simulink subsystem "rss_ComFaltDia"  (R2023a)
settings: Solver=VariableStepAuto  StartTime=0.0  StopTime=10.0  RelTol=1e-3
undefined symbols (not defined in the file): Cdbl_nMechSpdMaxVal, Cdbl_numComFramLosSmpNum, Cdbl_numDataExcdLimSmpNum, ENM_TYPE_FALT, Gs16_nMaxRefMechSpd_C, Gu16_ctComLosFaltConfCnt_C, Gu16_ctComLosFaltRcvyCnt_C, Gu16_ctComRolCntFaltConfCnt_C, Gu16_ctComRolCntFaltRcvyCnt_C, Gu16_ctCRCFaltConfCnt_C, Gu16_ctCRCFaltRcvyCnt_C, Gu16_ctMesgLngthFaltConfCnt_C, Gu16_ctMesgLngthFaltRcvyCnt_C, Gu8_ctComFramLosFaltJudgCnt_C, Gu8_ctDataExcdLimFaltJudgCnt_C, Gu8_RollingMax_C, Gu8_RollingMin_C
libraries: lib_debounce x7, simulink x5, lib_conversion x2, lib_fault_definiteness x1
settings Model: Creator=xiaoqiang.yuan  LastModifiedBy=xiaoqiang.yuan

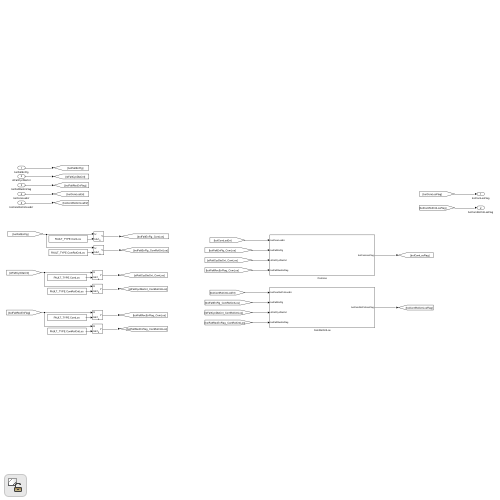
[thumbnail: Simulink's stored preview of the top-level diagram]
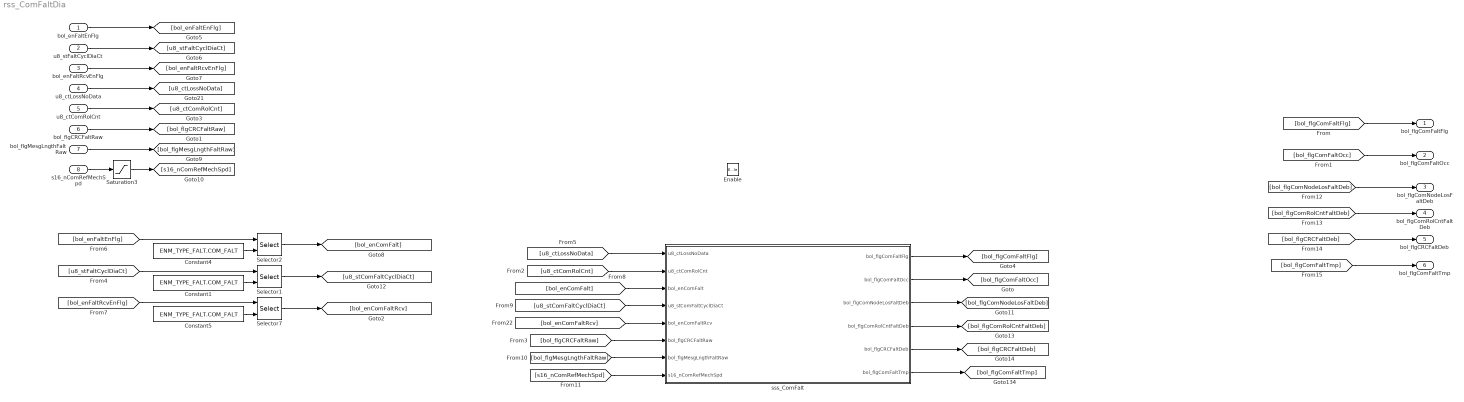
== system rss_ComFaltDia ==
  bol_enFaltEnFlg : Inport  OutDataTypeStr=boolean
  u8_stFaltCyclDiaCt : Inport  Port=2  OutDataTypeStr=uint8
  bol_enFaltRcvEnFlg : Inport  Port=3  OutDataTypeStr=boolean
  u8_ctLossNoData : Inport  Port=4  OutDataTypeStr=uint8
  u8_ctComRolCnt : Inport  Port=5  OutDataTypeStr=uint8
  bol_flgCRCFaltRaw : Inport  Port=6  OutDataTypeStr=boolean
  bol_flgMesgLngthFaltRaw : Inport  Port=7  OutDataTypeStr=boolean
  s16_nComRefMechSpd : Inport  Port=8  OutDataTypeStr=dt_Standardize_s16p15b0
  Enable : EnablePort
  Constant1 : Constant  Value=ENM_TYPE_FALT.COM_FALT
  Constant4 : Constant  Value=ENM_TYPE_FALT.COM_FALT
  Constant5 : Constant  Value=ENM_TYPE_FALT.COM_FALT
  Saturation3 : Saturate  UpperLimit=Cdbl_nMechSpdMaxVal  LowerLimit=-Cdbl_nMechSpdMaxVal
  Selector1 : Selector  IndexMode=Zero-based  InputPortWidth=Cdbl_numFaltDiaNum  IndexOptions=Index vector (port)  Indices=[1 3]  OutputSizes=1
  Selector2 : Selector  IndexMode=Zero-based  InputPortWidth=Cdbl_numFaltDiaNum  IndexOptions=Index vector (port)  Indices=[1 3]  OutputSizes=1
  Selector7 : Selector  IndexMode=Zero-based  InputPortWidth=Cdbl_numFaltDiaNum  IndexOptions=Index vector (port)  Indices=[1 3]  OutputSizes=1
  sss_ComFalt : Subsystem
  bol_flgComFaltFlg : Outport  OutDataTypeStr=boolean
  bol_flgComFaltOcc : Outport  Port=2  OutDataTypeStr=boolean
  bol_flgComNodeLosFaltDeb : Outport  Port=3  OutDataTypeStr=boolean
  bol_flgComRolCntFaltDeb : Outport  Port=4  OutDataTypeStr=boolean
  bol_flgCRCFaltDeb : Outport  Port=5  OutDataTypeStr=boolean
  bol_flgComFaltTmp : Outport  Port=6  OutDataTypeStr=boolean
  wires:
  [bol_flgComFaltFlg] -> bol_flgComFaltFlg/1
  [bol_flgComFaltOcc] -> bol_flgComFaltOcc/1
  [u8_stFaltCyclDiaCt] -> Selector1/1
  [bol_enFaltEnFlg] -> Selector2/1
  bol_enFaltEnFlg/1 -> [bol_enFaltEnFlg]
  bol_enFaltRcvEnFlg/1 -> [bol_enFaltRcvEnFlg]
  [u8_ctLossNoData] -> sss_ComFalt/1(u8_ctLossNoData)
  Constant1/1 -> Selector1/2
  [u8_stComFaltCyclDiaCt] -> sss_ComFalt/4(u8_stComFaltCyclDiaCt)
  [bol_enComFalt] -> sss_ComFalt/3(bol_enComFalt)
  Constant4/1 -> Selector2/2
  Constant5/1 -> Selector7/2
  Selector1/1 -> [u8_stComFaltCyclDiaCt]
  u8_ctLossNoData/1 -> [u8_ctLossNoData]
  Selector7/1 -> [bol_enComFaltRcv]
  [bol_enFaltRcvEnFlg] -> Selector7/1
  Selector2/1 -> [bol_enComFalt]
  [bol_enComFaltRcv] -> sss_ComFalt/5(bol_enComFaltRcv)
  u8_stFaltCyclDiaCt/1 -> [u8_stFaltCyclDiaCt]
  sss_ComFalt/1(bol_flgComFaltFlg) -> [bol_flgComFaltFlg]
  u8_ctComRolCnt/1 -> [u8_ctComRolCnt]
  [u8_ctComRolCnt] -> sss_ComFalt/2(u8_ctComRolCnt)
  sss_ComFalt/2(bol_flgComFaltOcc) -> [bol_flgComFaltOcc]
  bol_flgCRCFaltRaw/1 -> [bol_flgCRCFaltRaw]
  bol_flgMesgLngthFaltRaw/1 -> [bol_flgMesgLngthFaltRaw]
  s16_nComRefMechSpd/1 -> Saturation3/1
  [bol_flgCRCFaltRaw] -> sss_ComFalt/6(bol_flgCRCFaltRaw)
  [bol_flgMesgLngthFaltRaw] -> sss_ComFalt/7(bol_flgMesgLngthFaltRaw)
  [s16_nComRefMechSpd] -> sss_ComFalt/8(s16_nComRefMechSpd)
  Saturation3/1 -> [s16_nComRefMechSpd]
  [bol_flgCRCFaltDeb] -> bol_flgCRCFaltDeb/1
  [bol_flgComRolCntFaltDeb] -> bol_flgComRolCntFaltDeb/1
  [bol_flgComNodeLosFaltDeb] -> bol_flgComNodeLosFaltDeb/1
  sss_ComFalt/5(bol_flgCRCFaltDeb) -> [bol_flgCRCFaltDeb]
  sss_ComFalt/4(bol_flgComRolCntFaltDeb) -> [bol_flgComRolCntFaltDeb]
  sss_ComFalt/3(bol_flgComNodeLosFaltDeb) -> [bol_flgComNodeLosFaltDeb]
  [bol_flgComFaltTmp] -> bol_flgComFaltTmp/1
  sss_ComFalt/6(bol_flgComFaltTmp) -> [bol_flgComFaltTmp]

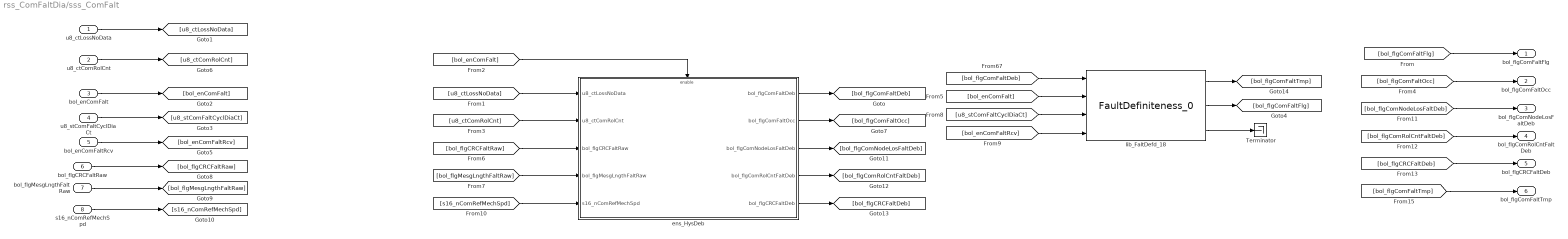
== system rss_ComFaltDia/sss_ComFalt ==
  u8_ctLossNoData : Inport
  u8_ctComRolCnt : Inport  Port=2
  bol_enComFalt : Inport  Port=3
  u8_stComFaltCyclDiaCt : Inport  Port=4
  bol_enComFaltRcv : Inport  Port=5
  bol_flgCRCFaltRaw : Inport  Port=6
  bol_flgMesgLngthFaltRaw : Inport  Port=7
  s16_nComRefMechSpd : Inport  Port=8
  Terminator : Terminator
  ens_HysDeb : Subsystem  Variant=on  VariantControlMode=label  VariantControl=Choice  LabelModeActiveChoice=GEELY_PROJECT
  lib_FaltDefd_18 : lib_fault_definiteness/FaultDefiniteness_0  lb_FaltWaitRecvCnt=0
  bol_flgComFaltFlg : Outport
  bol_flgComFaltOcc : Outport  Port=2
  bol_flgComNodeLosFaltDeb : Outport  Port=3
  bol_flgComRolCntFaltDeb : Outport  Port=4
  bol_flgCRCFaltDeb : Outport  Port=5
  bol_flgComFaltTmp : Outport  Port=6
  wires:
  [bol_flgComFaltTmp] -> bol_flgComFaltTmp/1
  ens_HysDeb/5(bol_flgCRCFaltDeb) -> [bol_flgCRCFaltDeb]
  ens_HysDeb/4(bol_flgComRolCntFaltDeb) -> [bol_flgComRolCntFaltDeb]
  ens_HysDeb/3(bol_flgComNodeLosFaltDeb) -> [bol_flgComNodeLosFaltDeb]
  [bol_flgCRCFaltDeb] -> bol_flgCRCFaltDeb/1
  [bol_flgComRolCntFaltDeb] -> bol_flgComRolCntFaltDeb/1
  [bol_flgComNodeLosFaltDeb] -> bol_flgComNodeLosFaltDeb/1
  ens_HysDeb/2(bol_flgComFaltOcc) -> [bol_flgComFaltOcc]
  ens_HysDeb/1(bol_flgComFaltDeb) -> [bol_flgComFaltDeb]
  [bol_enComFalt] -> ens_HysDeb/Enable
  [s16_nComRefMechSpd] -> ens_HysDeb/5(s16_nComRefMechSpd)
  [bol_flgMesgLngthFaltRaw] -> ens_HysDeb/4(bol_flgMesgLngthFaltRaw)
  [bol_flgCRCFaltRaw] -> ens_HysDeb/3(bol_flgCRCFaltRaw)
  [u8_ctComRolCnt] -> ens_HysDeb/2(u8_ctComRolCnt)
  [u8_ctLossNoData] -> ens_HysDeb/1(u8_ctLossNoData)
  bol_flgMesgLngthFaltRaw/1 -> [bol_flgMesgLngthFaltRaw]
  s16_nComRefMechSpd/1 -> [s16_nComRefMechSpd]
  bol_flgCRCFaltRaw/1 -> [bol_flgCRCFaltRaw]
  [bol_flgComFaltOcc] -> bol_flgComFaltOcc/1
  u8_ctComRolCnt/1 -> [u8_ctComRolCnt]
  lib_FaltDefd_18/1 -> [bol_flgComFaltTmp]
  lib_FaltDefd_18/2 -> [bol_flgComFaltFlg]
  lib_FaltDefd_18/3 -> Terminator/1
  bol_enComFaltRcv/1 -> [bol_enComFaltRcv]
  u8_stComFaltCyclDiaCt/1 -> [u8_stComFaltCyclDiaCt]
  bol_enComFalt/1 -> [bol_enComFalt]
  [bol_flgComFaltFlg] -> bol_flgComFaltFlg/1
  u8_ctLossNoData/1 -> [u8_ctLossNoData]
  [bol_enComFaltRcv] -> lib_FaltDefd_18/4
  [u8_stComFaltCyclDiaCt] -> lib_FaltDefd_18/3
  [bol_enComFalt] -> lib_FaltDefd_18/2
  [bol_flgComFaltDeb] -> lib_FaltDefd_18/1

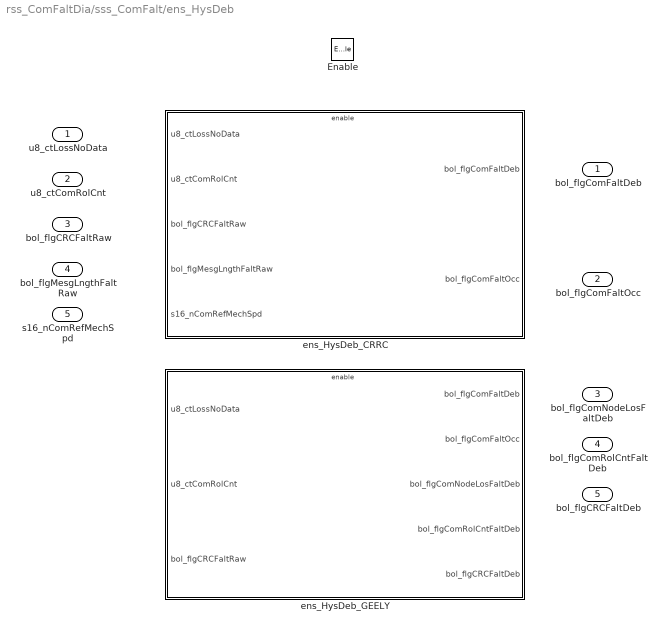
== system rss_ComFaltDia/sss_ComFalt/ens_HysDeb ==
  u8_ctLossNoData : Inport
  u8_ctComRolCnt : Inport  Port=2
  bol_flgCRCFaltRaw : Inport  Port=3
  bol_flgMesgLngthFaltRaw : Inport  Port=4
  s16_nComRefMechSpd : Inport  Port=5
  Enable : EnablePort
  ens_HysDeb_CRRC : Subsystem  VariantControl=CRRC_PROJECT
  ens_HysDeb_GEELY : Subsystem  VariantControl=GEELY_PROJECT
  bol_flgComFaltDeb : Outport
  bol_flgComFaltOcc : Outport  Port=2
  bol_flgComNodeLosFaltDeb : Outport  Port=3
  bol_flgComRolCntFaltDeb : Outport  Port=4
  bol_flgCRCFaltDeb : Outport  Port=5

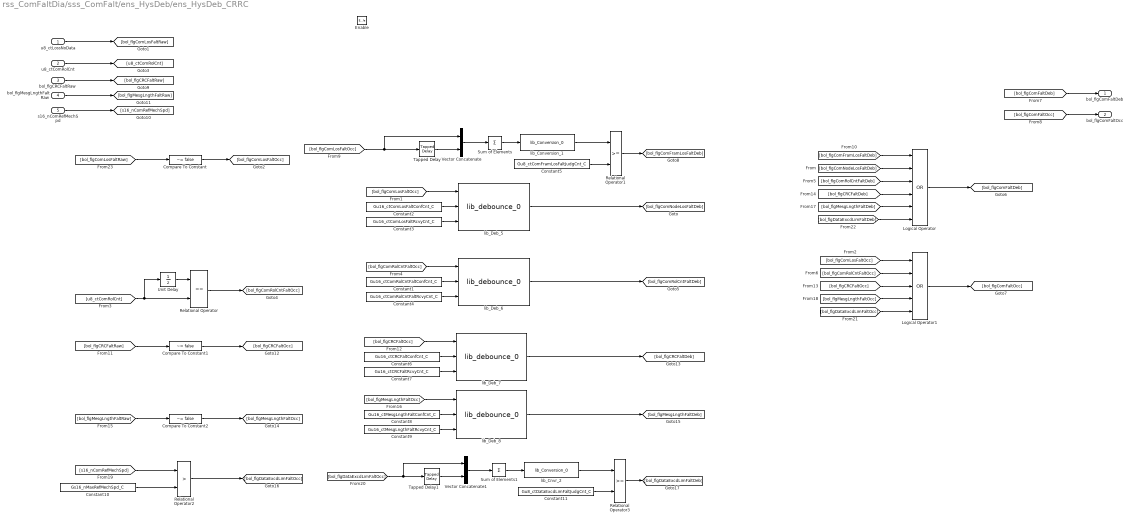
== system rss_ComFaltDia/sss_ComFalt/ens_HysDeb/ens_HysDeb_CRRC ==
  u8_ctLossNoData : Inport
  u8_ctComRolCnt : Inport  Port=2
  bol_flgCRCFaltRaw : Inport  Port=3
  bol_flgMesgLngthFaltRaw : Inport  Port=4
  s16_nComRefMechSpd : Inport  Port=5
  Enable : EnablePort
  Compare To Constant : simulink/Logic and Bit Operations/Compare To Constant  relop=~=  const=false  OutDataTypeStr=boolean
  Compare To Constant1 : simulink/Logic and Bit Operations/Compare To Constant  relop=~=  const=false  OutDataTypeStr=boolean
  Compare To Constant2 : simulink/Logic and Bit Operations/Compare To Constant  relop=~=  const=false  OutDataTypeStr=boolean
  Constant1 : Constant  Value=Gu16_ctComRolCntFaltConfCnt_C
  Constant10 : Constant  Value=Gs16_nMaxRefMechSpd_C
  Constant11 : Constant  Value=Gu8_ctDataExcdLimFaltJudgCnt_C
  Constant2 : Constant  Value=Gu16_ctComLosFaltConfCnt_C
  Constant3 : Constant  Value=Gu16_ctComLosFaltRcvyCnt_C
  Constant4 : Constant  Value=Gu16_ctComRolCntFaltRcvyCnt_C
  Constant5 : Constant  Value=Gu8_ctComFramLosFaltJudgCnt_C
  Constant6 : Constant  Value=Gu16_ctCRCFaltConfCnt_C
  Constant7 : Constant  Value=Gu16_ctCRCFaltRcvyCnt_C
  Constant8 : Constant  Value=Gu16_ctMesgLngthFaltConfCnt_C
  Constant9 : Constant  Value=Gu16_ctMesgLngthFaltRcvyCnt_C
  Logical Operator : Logic  Operator=OR  Inputs=6  AllPortsSameDT=off  OutDataTypeStr=boolean
  Logical Operator1 : Logic  Operator=OR  Inputs=5  AllPortsSameDT=off  OutDataTypeStr=boolean
  Relational Operator : RelationalOperator  Operator===  OutDataTypeStr=boolean  RndMeth=Simplest  InputSameDT=off
  Relational Operator1 : RelationalOperator  OutDataTypeStr=boolean  RndMeth=Simplest  InputSameDT=off
  Relational Operator2 : RelationalOperator  Operator=>  OutDataTypeStr=boolean  RndMeth=Simplest  InputSameDT=off
  Relational Operator3 : RelationalOperator  OutDataTypeStr=boolean  RndMeth=Simplest  InputSameDT=off
  Sum of Elements : Sum  Inputs=+  OutDataTypeStr=Inherit: Inherit via back propagation  RndMeth=Simplest
  Sum of Elements1 : Sum  Inputs=+  OutDataTypeStr=Inherit: Inherit via back propagation  RndMeth=Simplest
  Tapped Delay : simulink/Discrete/Tapped Delay  vinit=0  samptime=-1  NumDelays=Cdbl_numComFramLosSmpNum-1  DelayOrder=Oldest  includeCurrent=off
  Tapped Delay1 : simulink/Discrete/Tapped Delay  vinit=0  samptime=-1  NumDelays=Cdbl_numDataExcdLimSmpNum-1  DelayOrder=Oldest  includeCurrent=off
  Unit Delay : UnitDelay  SampleTime=-1  HasFrameUpgradeWarning=on
  Vector Concatenate : Concatenate
  Vector Concatenate1 : Concatenate
  lib_Cnvr_2 : lib_conversion/lib_Conversion_0  lb_parDataType=uint8  lb_parOutpMaxVal=[]  lb_parOutpMinVal=[]  lb_parSatFlag=off
  lib_Conversion_1 : lib_conversion/lib_Conversion_0  lb_parDataType=uint8  lb_parOutpMaxVal=[]  lb_parOutpMinVal=[]  lb_parSatFlag=off
  lib_Deb_{5..8} (4 alike) : lib_debounce/lib_debounce_0
  bol_flgComFaltDeb : Outport
  bol_flgComFaltOcc : Outport  Port=2
  wires:
  [bol_flgDataExcdLimFaltOcc] -> Logical Operator1/5
  [bol_flgMesgLngthFaltOcc] -> Logical Operator1/4
  [bol_flgDataExcdLimFaltDeb] -> Logical Operator/6
  [bol_flgMesgLngthFaltDeb] -> Logical Operator/5
  Relational Operator3/1 -> [bol_flgDataExcdLimFaltDeb]
  Constant11/1 -> Relational Operator3/2
  lib_Cnvr_2/1 -> Relational Operator3/1
  Tapped Delay1/1 -> Vector Concatenate1/2
  Vector Concatenate1/1 -> Sum of Elements1/1
  [bol_flgDataExcdLimFaltOcc] -> Tapped Delay1/1, Vector Concatenate1/1
  Sum of Elements1/1 -> lib_Cnvr_2/1
  Relational Operator2/1 -> [bol_flgDataExcdLimFaltOcc]
  Constant10/1 -> Relational Operator2/2
  [s16_nComRefMechSpd] -> Relational Operator2/1
  lib_Deb_8/1 -> [bol_flgMesgLngthFaltDeb]
  [bol_flgMesgLngthFaltOcc] -> lib_Deb_8/1
  Constant8/1 -> lib_Deb_8/2
  Constant9/1 -> lib_Deb_8/3
  Compare To Constant2/1 -> [bol_flgMesgLngthFaltOcc]
  [bol_flgMesgLngthFaltRaw] -> Compare To Constant2/1
  [bol_flgCRCFaltOcc] -> Logical Operator1/3
  [bol_flgComRolCntFaltOcc] -> Logical Operator1/2
  [bol_flgComLosFaltOcc] -> Logical Operator1/1
  [bol_flgComFramLosFaltDeb] -> Logical Operator/1
  [bol_flgComNodeLosFaltDeb] -> Logical Operator/2
  [bol_flgComRolCntFaltDeb] -> Logical Operator/3
  [bol_flgCRCFaltDeb] -> Logical Operator/4
  lib_Deb_7/1 -> [bol_flgCRCFaltDeb]
  Constant7/1 -> lib_Deb_7/3
  Constant6/1 -> lib_Deb_7/2
  [bol_flgCRCFaltOcc] -> lib_Deb_7/1
  Compare To Constant1/1 -> [bol_flgCRCFaltOcc]
  [bol_flgCRCFaltRaw] -> Compare To Constant1/1
  s16_nComRefMechSpd/1 -> [s16_nComRefMechSpd]
  bol_flgCRCFaltRaw/1 -> [bol_flgCRCFaltRaw]
  bol_flgMesgLngthFaltRaw/1 -> [bol_flgMesgLngthFaltRaw]
  Relational Operator1/1 -> [bol_flgComFramLosFaltDeb]
  Constant5/1 -> Relational Operator1/2
  lib_Conversion_1/1 -> Relational Operator1/1
  Sum of Elements/1 -> lib_Conversion_1/1
  [bol_flgComLosFaltOcc] -> Tapped Delay/1, Vector Concatenate/1
  Tapped Delay/1 -> Vector Concatenate/2
  Vector Concatenate/1 -> Sum of Elements/1
  [bol_flgComFaltOcc] -> bol_flgComFaltOcc/1
  Logical Operator1/1 -> [bol_flgComFaltOcc]
  Logical Operator/1 -> [bol_flgComFaltDeb]
  lib_Deb_6/1 -> [bol_flgComRolCntFaltDeb]
  [bol_flgComRolCntFaltOcc] -> lib_Deb_6/1
  Constant1/1 -> lib_Deb_6/2
  Constant4/1 -> lib_Deb_6/3
  Relational Operator/1 -> [bol_flgComRolCntFaltOcc]
  Unit Delay/1 -> Relational Operator/1
  [u8_ctComRolCnt] -> Unit Delay/1, Relational Operator/2
  u8_ctComRolCnt/1 -> [u8_ctComRolCnt]
  [bol_flgComLosFaltOcc] -> lib_Deb_5/1
  Compare To Constant/1 -> [bol_flgComLosFaltOcc]
  [bol_flgComLosFaltRaw] -> Compare To Constant/1
  lib_Deb_5/1 -> [bol_flgComNodeLosFaltDeb]
  u8_ctLossNoData/1 -> [bol_flgComLosFaltRaw]
  [bol_flgComFaltDeb] -> bol_flgComFaltDeb/1
  Constant3/1 -> lib_Deb_5/3
  Constant2/1 -> lib_Deb_5/2

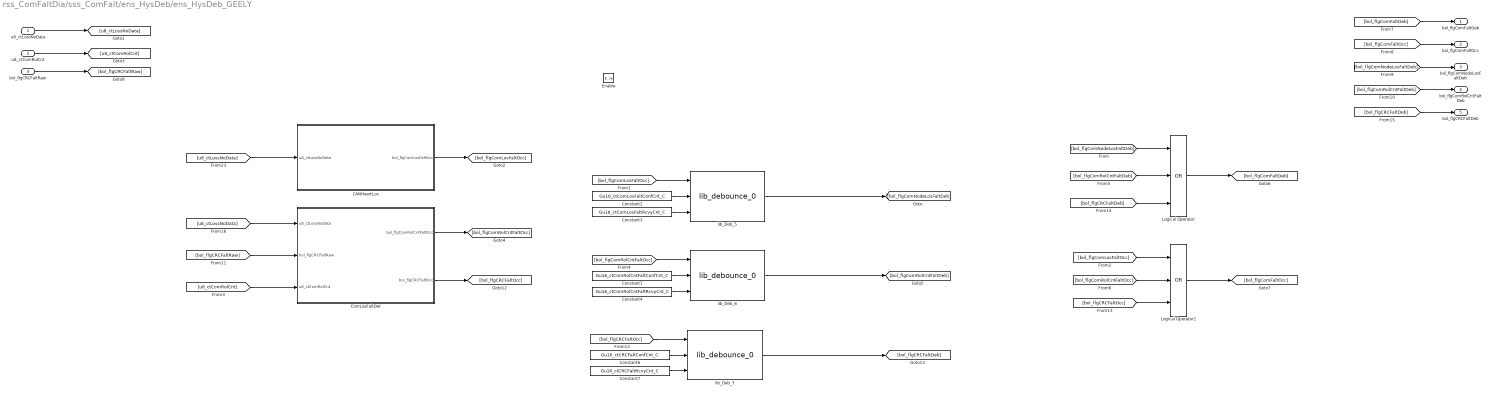
== system rss_ComFaltDia/sss_ComFalt/ens_HysDeb/ens_HysDeb_GEELY ==
  u8_ctLossNoData : Inport
  u8_ctComRolCnt : Inport  Port=2
  bol_flgCRCFaltRaw : Inport  Port=3
  Enable : EnablePort
  CANHeartLos : Subsystem  RTWFcnName=CANHeartLosCheck
      settings: RTWSystemCode=Nonreusable function  RTWFcnNameOpts=User specified
  ComLosFaltDet : Subsystem
  Constant1 : Constant  Value=Gu16_ctComRolCntFaltConfCnt_C
  Constant2 : Constant  Value=Gu16_ctComLosFaltConfCnt_C
  Constant3 : Constant  Value=Gu16_ctComLosFaltRcvyCnt_C
  Constant4 : Constant  Value=Gu16_ctComRolCntFaltRcvyCnt_C
  Constant6 : Constant  Value=Gu16_ctCRCFaltConfCnt_C
  Constant7 : Constant  Value=Gu16_ctCRCFaltRcvyCnt_C
  Logical Operator : Logic  Operator=OR  Inputs=3  AllPortsSameDT=off  OutDataTypeStr=boolean
  Logical Operator1 : Logic  Operator=OR  Inputs=3  AllPortsSameDT=off  OutDataTypeStr=boolean
  lib_Deb_5 : lib_debounce/lib_debounce_0
  lib_Deb_6 : lib_debounce/lib_debounce_0
  lib_Deb_7 : lib_debounce/lib_debounce_0
  bol_flgComFaltDeb : Outport
  bol_flgComFaltOcc : Outport  Port=2
  bol_flgComNodeLosFaltDeb : Outport  Port=3
  bol_flgComRolCntFaltDeb : Outport  Port=4
  bol_flgCRCFaltDeb : Outport  Port=5
  wires:
  [u8_ctLossNoData] -> ComLosFaltDet/1(u8_ctLossNoData)
  CANHeartLos/1(bol_flgComLosFaltOcc) -> [bol_flgComLosFaltOcc]
  [u8_ctLossNoData] -> CANHeartLos/1(u8_ctLossNoData)
  ComLosFaltDet/1(bol_flgComRolCntFaltOcc) -> [bol_flgComRolCntFaltOcc]
  ComLosFaltDet/2(bol_flgCRCFaltOcc) -> [bol_flgCRCFaltOcc]
  [bol_flgCRCFaltRaw] -> ComLosFaltDet/2(bol_flgCRCFaltRaw)
  [u8_ctComRolCnt] -> ComLosFaltDet/3(u8_ctComRolCnt)
  [bol_flgCRCFaltDeb] -> bol_flgCRCFaltDeb/1
  [bol_flgComRolCntFaltDeb] -> bol_flgComRolCntFaltDeb/1
  [bol_flgComNodeLosFaltDeb] -> bol_flgComNodeLosFaltDeb/1
  [bol_flgCRCFaltOcc] -> Logical Operator1/3
  [bol_flgComRolCntFaltOcc] -> Logical Operator1/2
  [bol_flgComLosFaltOcc] -> Logical Operator1/1
  [bol_flgComNodeLosFaltDeb] -> Logical Operator/1
  [bol_flgComRolCntFaltDeb] -> Logical Operator/2
  [bol_flgCRCFaltDeb] -> Logical Operator/3
  lib_Deb_7/1 -> [bol_flgCRCFaltDeb]
  Constant7/1 -> lib_Deb_7/3
  Constant6/1 -> lib_Deb_7/2
  [bol_flgCRCFaltOcc] -> lib_Deb_7/1
  bol_flgCRCFaltRaw/1 -> [bol_flgCRCFaltRaw]
  [bol_flgComFaltOcc] -> bol_flgComFaltOcc/1
  Logical Operator1/1 -> [bol_flgComFaltOcc]
  Logical Operator/1 -> [bol_flgComFaltDeb]
  lib_Deb_6/1 -> [bol_flgComRolCntFaltDeb]
  [bol_flgComRolCntFaltOcc] -> lib_Deb_6/1
  Constant1/1 -> lib_Deb_6/2
  Constant4/1 -> lib_Deb_6/3
  u8_ctComRolCnt/1 -> [u8_ctComRolCnt]
  [bol_flgComLosFaltOcc] -> lib_Deb_5/1
  lib_Deb_5/1 -> [bol_flgComNodeLosFaltDeb]
  u8_ctLossNoData/1 -> [u8_ctLossNoData]
  [bol_flgComFaltDeb] -> bol_flgComFaltDeb/1
  Constant3/1 -> lib_Deb_5/3
  Constant2/1 -> lib_Deb_5/2

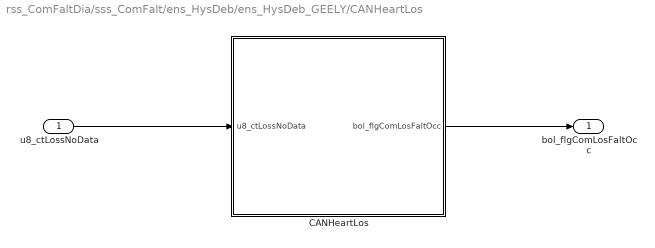
== system rss_ComFaltDia/sss_ComFalt/ens_HysDeb/ens_HysDeb_GEELY/CANHeartLos ==
  u8_ctLossNoData : Inport
  CANHeartLos : Subsystem
  bol_flgComLosFaltOcc : Outport
  wires:
  CANHeartLos/1(bol_flgComLosFaltOcc) -> bol_flgComLosFaltOcc/1
  u8_ctLossNoData/1 -> CANHeartLos/1(u8_ctLossNoData)

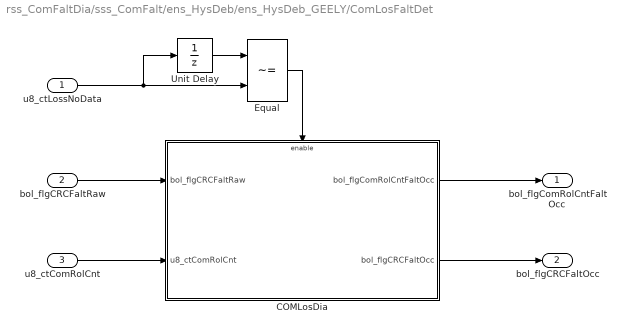
== system rss_ComFaltDia/sss_ComFalt/ens_HysDeb/ens_HysDeb_GEELY/ComLosFaltDet ==
  u8_ctLossNoData : Inport
  bol_flgCRCFaltRaw : Inport  Port=2
  u8_ctComRolCnt : Inport  Port=3
  COMLosDia : Subsystem  TreatAsAtomicUnit=on  RTWFcnName=CANSigLosCheck
      settings: RTWSystemCode=Nonreusable function  RTWFcnNameOpts=User specified
  Equal : RelationalOperator  Operator=~=  OutDataTypeStr=boolean  RndMeth=Simplest  InputSameDT=off
  Unit Delay : UnitDelay  SampleTime=-1  HasFrameUpgradeWarning=on
  bol_flgComRolCntFaltOcc : Outport
  bol_flgCRCFaltOcc : Outport  Port=2
  wires:
  u8_ctLossNoData/1 -> Equal/2, Unit Delay/1
  Unit Delay/1 -> Equal/1
  Equal/1 -> COMLosDia/Enable
  COMLosDia/2(bol_flgCRCFaltOcc) -> bol_flgCRCFaltOcc/1
  bol_flgCRCFaltRaw/1 -> COMLosDia/1(bol_flgCRCFaltRaw)
  COMLosDia/1(bol_flgComRolCntFaltOcc) -> bol_flgComRolCntFaltOcc/1
  u8_ctComRolCnt/1 -> COMLosDia/2(u8_ctComRolCnt)

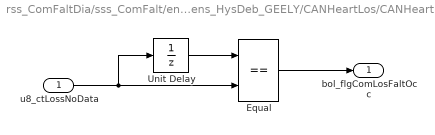
== system rss_ComFaltDia/sss_ComFalt/ens_HysDeb/ens_HysDeb_GEELY/CANHeartLos/CANHeartLos ==
  u8_ctLossNoData : Inport
  Equal : RelationalOperator  Operator===  OutDataTypeStr=boolean  RndMeth=Simplest  InputSameDT=off
  Unit Delay : UnitDelay  SampleTime=-1  HasFrameUpgradeWarning=on
  bol_flgComLosFaltOcc : Outport
  wires:
  Equal/1 -> bol_flgComLosFaltOcc/1
  Unit Delay/1 -> Equal/1
  u8_ctLossNoData/1 -> Unit Delay/1, Equal/2

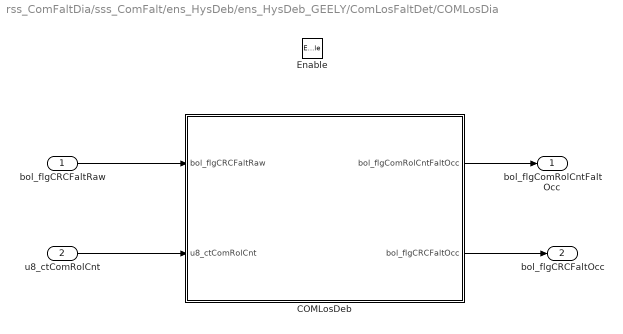
== system rss_ComFaltDia/sss_ComFalt/ens_HysDeb/ens_HysDeb_GEELY/ComLosFaltDet/COMLosDia ==
  bol_flgCRCFaltRaw : Inport
  u8_ctComRolCnt : Inport  Port=2
  Enable : EnablePort
  COMLosDeb : Subsystem
  bol_flgComRolCntFaltOcc : Outport  InitialOutput=0
  bol_flgCRCFaltOcc : Outport  Port=2  InitialOutput=0
  wires:
  COMLosDeb/2(bol_flgCRCFaltOcc) -> bol_flgCRCFaltOcc/1
  COMLosDeb/1(bol_flgComRolCntFaltOcc) -> bol_flgComRolCntFaltOcc/1
  bol_flgCRCFaltRaw/1 -> COMLosDeb/1(bol_flgCRCFaltRaw)
  u8_ctComRolCnt/1 -> COMLosDeb/2(u8_ctComRolCnt)

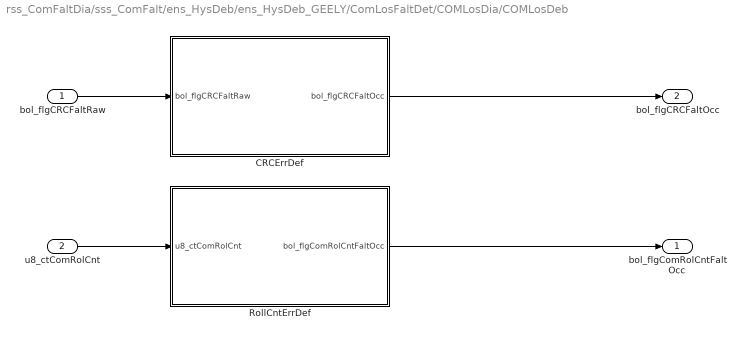
== system rss_ComFaltDia/sss_ComFalt/ens_HysDeb/ens_HysDeb_GEELY/ComLosFaltDet/COMLosDia/COMLosDeb ==
  bol_flgCRCFaltRaw : Inport
  u8_ctComRolCnt : Inport  Port=2
  CRCErrDef : Subsystem
  RollCntErrDef : Subsystem
  bol_flgComRolCntFaltOcc : Outport  OutputWhenDisabled=reset  InitialOutput=0
  bol_flgCRCFaltOcc : Outport  Port=2  OutputWhenDisabled=reset  InitialOutput=0
  wires:
  RollCntErrDef/1(bol_flgComRolCntFaltOcc) -> bol_flgComRolCntFaltOcc/1
  CRCErrDef/1(bol_flgCRCFaltOcc) -> bol_flgCRCFaltOcc/1
  u8_ctComRolCnt/1 -> RollCntErrDef/1(u8_ctComRolCnt)
  bol_flgCRCFaltRaw/1 -> CRCErrDef/1(bol_flgCRCFaltRaw)

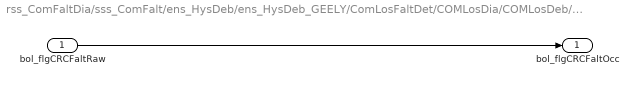
== system rss_ComFaltDia/sss_ComFalt/ens_HysDeb/ens_HysDeb_GEELY/ComLosFaltDet/COMLosDia/COMLosDeb/CRCErrDef ==
  bol_flgCRCFaltRaw : Inport
  bol_flgCRCFaltOcc : Outport
  wires:
  bol_flgCRCFaltRaw/1 -> bol_flgCRCFaltOcc/1

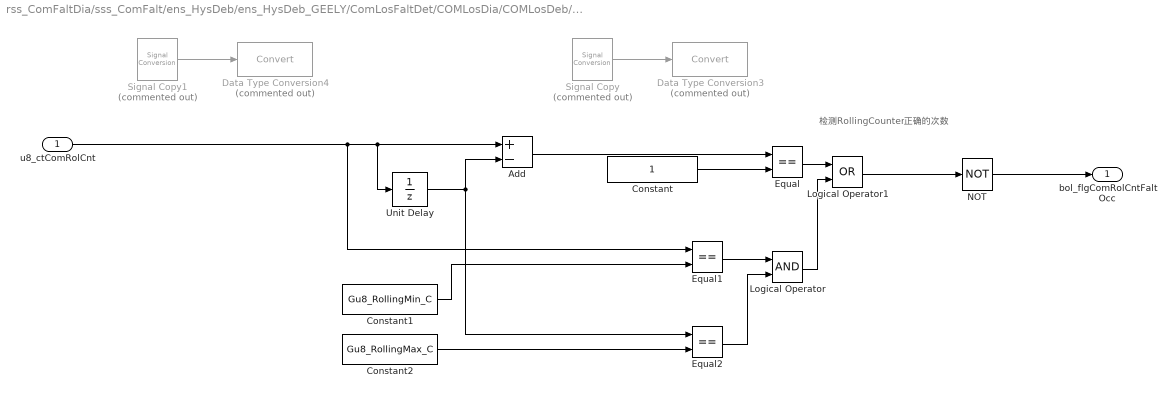
== system rss_ComFaltDia/sss_ComFalt/ens_HysDeb/ens_HysDeb_GEELY/ComLosFaltDet/COMLosDia/COMLosDeb/RollCntErrDef ==
  note: 检测RollingCounter正确的次数
  u8_ctComRolCnt : Inport
  Add : Sum  Inputs=+-
  Constant : Constant  OutDataTypeStr=uint8
  Constant1 : Constant  Value=Gu8_RollingMin_C  OutDataTypeStr=uint8
  Constant2 : Constant  Value=Gu8_RollingMax_C  OutDataTypeStr=uint8
  Data Type Conversion3 : DataTypeConversion  Commented=on  SaturateOnIntegerOverflow=off  RndMeth=Floor
  Data Type Conversion4 : DataTypeConversion  Commented=on  SaturateOnIntegerOverflow=off  RndMeth=Floor
  Equal : RelationalOperator  Operator===  OutDataTypeStr=boolean  RndMeth=Simplest  InputSameDT=off
  Equal1 : RelationalOperator  Operator===  OutDataTypeStr=boolean  RndMeth=Simplest  InputSameDT=off
  Equal2 : RelationalOperator  Operator===  OutDataTypeStr=boolean  RndMeth=Simplest  InputSameDT=off
  Logical Operator : Logic  AllPortsSameDT=off  OutDataTypeStr=boolean
  Logical Operator1 : Logic  Operator=OR  AllPortsSameDT=off  OutDataTypeStr=boolean
  NOT : Logic  Operator=NOT  AllPortsSameDT=off  OutDataTypeStr=boolean
  Signal Copy : SignalConversion  Commented=on  OverrideOpt=off
  Signal Copy1 : SignalConversion  Commented=on  OverrideOpt=off
  Unit Delay : UnitDelay  SampleTime=-1  HasFrameUpgradeWarning=on
  bol_flgComRolCntFaltOcc : Outport
  wires:
  Signal Copy1/1 -> Data Type Conversion4/1
  Add/1 -> Equal/1
  NOT/1 -> bol_flgComRolCntFaltOcc/1
  Signal Copy/1 -> Data Type Conversion3/1
  Constant/1 -> Equal/2
  Unit Delay/1 -> Equal2/1, Add/2
  Equal/1 -> Logical Operator1/1
  u8_ctComRolCnt/1 -> Equal1/1, Unit Delay/1, Add/1
  Constant1/1 -> Equal1/2
  Equal1/1 -> Logical Operator/1
  Constant2/1 -> Equal2/2
  Equal2/1 -> Logical Operator/2
  Logical Operator/1 -> Logical Operator1/2
  Logical Operator1/1 -> NOT/1
